simulink model "CP_SFC_Lin_b_n9558292"  (R2018a)
settings: Solver=ode4  StartTime=0.0  StopTime=10.0  FixedStep=0.02  RelTol=1e-3
values from neighbouring files (symbols this model uses):
  g = 9.81    [CP_SFC_Lin_b_MainFile_n9558292.m]
  Kb = place(Ab,Bb,Pb)    [CP_SFC_Lin_b_MainFile_n9558292.m]
  l = 0.2    [CP_SFC_Lin_b_MainFile_n9558292.m]
  m = 0.15    [CP_SFC_Lin_b_MainFile_n9558292.m]
  Mc = 0.4    [CP_SFC_Lin_b_MainFile_n9558292.m]
  x10 = 0.4    [CP_SFC_Lin_b_MainFile_n9558292.m]
  x20 = deg2rad(200)    [CP_SFC_Lin_b_MainFile_n9558292.m]
  x2_bar = pi    (= 3.14159265359)    [CP_SFC_Lin_b_MainFile_n9558292.m]
  x30 = 0    [CP_SFC_Lin_b_MainFile_n9558292.m]
  x40 = 0    [CP_SFC_Lin_b_MainFile_n9558292.m]
undefined symbols (not defined in the file or in its folder): u_bar
settings Model: Creator=haidarobeid  LastModifiedBy=haidarobeid

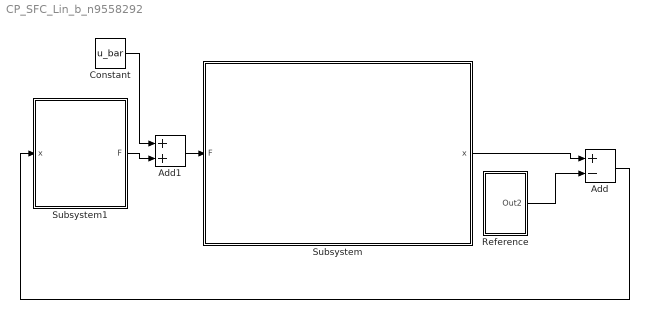
== system CP_SFC_Lin_b_n9558292 ==
  Add : Sum  Inputs=+-
  Add1 : Sum
  Constant : Constant  Value=u_bar
  Reference : Subsystem
  Subsystem : Subsystem
  Subsystem1 : Subsystem
  wires:
  Subsystem/1(x) -> Add/1
  Add/1 -> Subsystem1/1(x)
  Reference/1(Out2) -> Add/2
  Add1/1 -> Subsystem/1(F)
  Subsystem1/1(F) -> Add1/2
  Constant/1 -> Add1/1

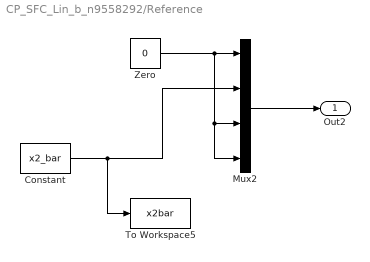
== system CP_SFC_Lin_b_n9558292/Reference ==
  Constant : Constant  Value=x2_bar
  Mux2 : Mux
  To Workspace5 : ToWorkspace  VariableName=x2bar  SaveFormat=Timeseries  SampleTime=-1
  Zero : Constant  Value=0
  Out2 : Outport
  wires:
  Mux2/1 -> Out2/1
  Constant/1 -> To Workspace5/1, Mux2/2
  Zero/1 -> Mux2/4, Mux2/3, Mux2/1

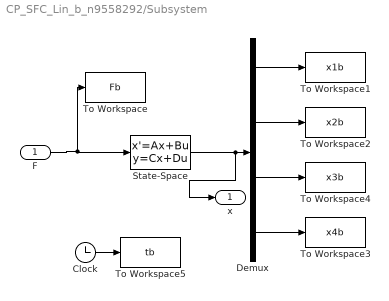
== system CP_SFC_Lin_b_n9558292/Subsystem ==
  F : Inport
  Clock : Clock
  Demux : Demux
  State-Space : StateSpace  A=[0,0,1,0;0,0,0,1;0,-(m*g/Mc),0,0;0,g*(Mc+m)/(l*Mc),0,0]  B=[0;0;1/Mc;1/(l*Mc)]  C=eye(4)  D=[0; 0; 0 ;0]  InitialCondition=[x10;x20;x30;x40]
  To Workspace : ToWorkspace  VariableName=Fb  SampleTime=-1
  To Workspace1 : ToWorkspace  VariableName=x1b  SampleTime=-1
  To Workspace2 : ToWorkspace  VariableName=x2b  SampleTime=-1
  To Workspace3 : ToWorkspace  VariableName=x4b  SampleTime=-1
  To Workspace4 : ToWorkspace  VariableName=x3b  SampleTime=-1
  To Workspace5 : ToWorkspace  VariableName=tb  SampleTime=-1
  x : Outport
  wires:
  Demux/3 -> To Workspace4/1
  Demux/2 -> To Workspace2/1
  Demux/4 -> To Workspace3/1
  State-Space/1 -> Demux/1, x/1
  F/1 -> State-Space/1, To Workspace/1
  Demux/1 -> To Workspace1/1
  Clock/1 -> To Workspace5/1

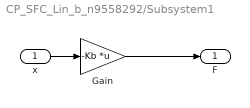
== system CP_SFC_Lin_b_n9558292/Subsystem1 ==
  x : Inport
  Gain : Gain  Gain=-Kb  Multiplication=Matrix(K*u)
  F : Outport
  wires:
  Gain/1 -> F/1
  x/1 -> Gain/1
